simulink model "Constant_Gain_Control_Simulation"  (R2018b)
settings: Solver=ode4  StartTime=0.0  StopTime=500  FixedStep=1e-3  RelTol=1e-3
settings Model: Creator=auralius  LastModifiedBy=auralius

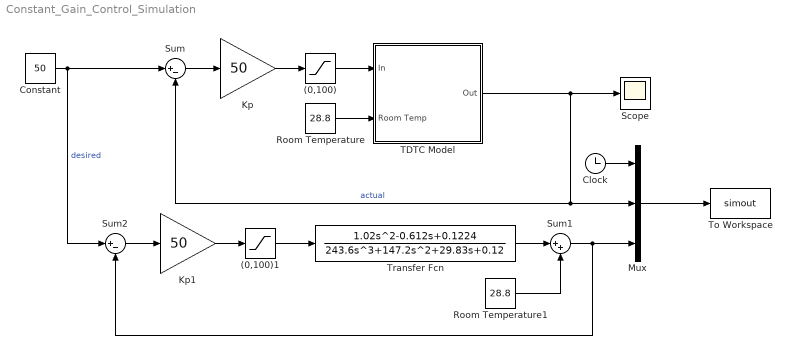
== system Constant_Gain_Control_Simulation ==
  (0,100) : Saturate  UpperLimit=100  LowerLimit=0
  (0,100)1 : Saturate  UpperLimit=100  LowerLimit=0
  Clock : Clock
  Constant : Constant  Value=50
  Kp : Gain  Gain=50
  Kp1 : Gain  Gain=50
  Mux : Mux  Inputs=3
  Room Temperature : Constant  Value=28.8
  Room Temperature1 : Constant  Value=28.8
  Scope : Scope
  Sum : Sum  Inputs=|+-
  Sum1 : Sum  Inputs=|++
  Sum2 : Sum  Inputs=|+-
  TDTC Model : Subsystem
  To Workspace : ToWorkspace  VariableName=simout  SampleTime=-1
  Transfer Fcn : TransferFcn  Numerator=[1.02 -0.612 0.1224]  Denominator=[243.6 147.2 29.83 0.12]
  wires:
  Mux/1 -> To Workspace/1
  Clock/1 -> Mux/1
  TDTC Model/1(Out) -> Scope/1, Mux/2, Sum/2  "actual"
  Sum/1 -> Kp/1
  Constant/1 -> Sum2/1, Sum/1  "desired"
  Kp/1 -> (0,100)/1
  (0,100)/1 -> TDTC Model/1(In)
  Room Temperature/1 -> TDTC Model/2(Room Temp)
  Room Temperature1/1 -> Sum1/2
  (0,100)1/1 -> Transfer Fcn/1
  Sum2/1 -> Kp1/1
  Kp1/1 -> (0,100)1/1
  Transfer Fcn/1 -> Sum1/1
  Sum1/1 -> Sum2/2, Mux/3

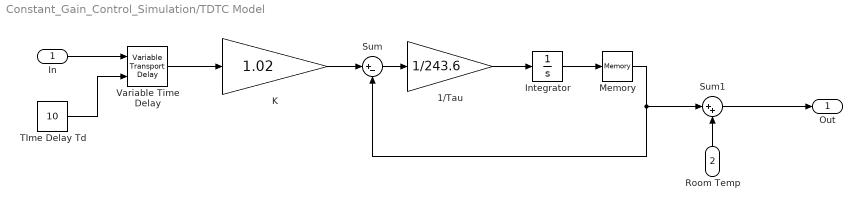
== system Constant_Gain_Control_Simulation/TDTC Model ==
  In : Inport
  Room Temp : Inport  Port=2
  1/Tau : Gain  Gain=1/243.6
  Integrator : Integrator
  K : Gain  Gain=1.02
  Memory : Memory
  Sum : Sum  Inputs=|+-
  Sum1 : Sum  Inputs=|++
  TIme Delay Td : Constant  Value=10
  Variable Time Delay : VariableTransportDelay  MaximumDelay=50
  Out : Outport
  wires:
  K/1 -> Sum/1
  Memory/1 -> Sum/2, Sum1/1
  In/1 -> Variable Time Delay/1
  Sum/1 -> 1/Tau/1
  Integrator/1 -> Memory/1
  Variable Time Delay/1 -> K/1
  Sum1/1 -> Out/1
  TIme Delay Td/1 -> Variable Time Delay/2
  1/Tau/1 -> Integrator/1
  Room Temp/1 -> Sum1/2
